simulink model "Modell_Entkopplung"  (R2025b)
settings: Solver=VariableStepAuto  StartTime=0.0  StopTime=10.0  RelTol=1e-3
values from neighbouring files (symbols this model uses):
  K1 = 4    [Modell_Entkopplung_Skript.m]
  K2 = 1    [Modell_Entkopplung_Skript.m]
  K3 = 3    [Modell_Entkopplung_Skript.m]
  K4 = 1    [Modell_Entkopplung_Skript.m]
  K5 = 1    [Modell_Entkopplung_Skript.m]
  K6 = 1    [Modell_Entkopplung_Skript.m]
  T1 = 1    [Modell_Entkopplung_Skript.m]
  T2 = 2    [Modell_Entkopplung_Skript.m]
  T3 = 1    [Modell_Entkopplung_Skript.m]
  T4 = 1    [Modell_Entkopplung_Skript.m]
  T5 = 1    [Modell_Entkopplung_Skript.m]
settings Model: Creator=ezech  LastModifiedBy=ezech

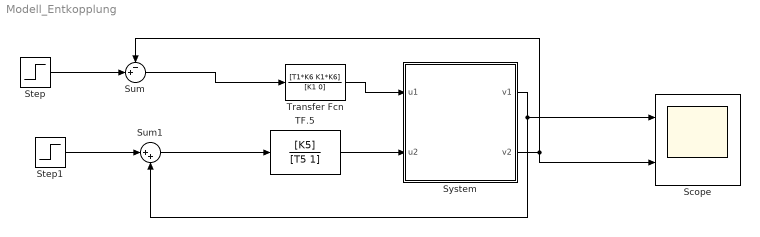
== system Modell_Entkopplung ==
  Scope : Scope  NumInputPorts=2
      settings: ActiveDisplayYMinimum=-1.0016844867769303  ActiveDisplayYMaximum=9.0151603809923753
  Step : Step  Time=0  SampleTime=0
  Step1 : Step  Time=0  After=0  SampleTime=0
  Sum : Sum  Inputs=-+|
  Sum1 : Sum  Inputs=|++
  System : Subsystem
  TF.5 : TransferFcn  Numerator=[K5]  Denominator=[T5 1]
  Transfer Fcn : TransferFcn  Numerator=[T1*K6 K1*K6]  Denominator=[K1 0]
  wires:
  Transfer Fcn/1 -> System/1(u1)
  TF.5/1 -> System/2(u2)
  Step/1 -> Sum/2
  System/2(v2) -> Sum/1, Scope/2
  Sum/1 -> Transfer Fcn/1
  Sum1/1 -> TF.5/1
  Step1/1 -> Sum1/1
  System/1(v1) -> Sum1/2, Scope/1

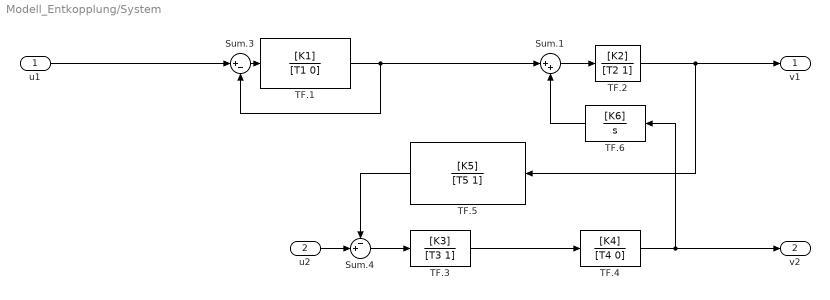
== system Modell_Entkopplung/System ==
  u1 : Inport
  u2 : Inport  Port=2
  Sum.1 : Sum  Inputs=|++  InputSameDT=on  SaturateOnIntegerOverflow=on  OutDataTypeStr=Inherit: Same as first input
  Sum.3 : Sum  Inputs=|+-  InputSameDT=on  SaturateOnIntegerOverflow=on  OutDataTypeStr=Inherit: Same as first input
  Sum.4 : Sum  Inputs=-+|  InputSameDT=on  SaturateOnIntegerOverflow=on  OutDataTypeStr=Inherit: Same as first input
  TF.1 : TransferFcn  Numerator=[K1]  Denominator=[T1 0]
  TF.2 : TransferFcn  Numerator=[K2]  Denominator=[T2 1]
  TF.3 : TransferFcn  Numerator=[K3]  Denominator=[T3 1]
  TF.4 : TransferFcn  Numerator=[K4]  Denominator=[T4 0]
  TF.5 : TransferFcn  Numerator=[K5]  Denominator=[T5 1]
  TF.6 : TransferFcn  Numerator=[K6]  Denominator=[1 0]
  v1 : Outport
  v2 : Outport  Port=2
  wires:
  TF.2/1 -> v1/1, TF.5/1
  TF.4/1 -> v2/1, TF.6/1
  TF.1/1 -> Sum.3/2, Sum.1/1
  Sum.1/1 -> TF.2/1
  TF.3/1 -> TF.4/1
  Sum.4/1 -> TF.3/1
  u2/1 -> Sum.4/2
  TF.5/1 -> Sum.4/1
  Sum.3/1 -> TF.1/1
  u1/1 -> Sum.3/1
  TF.6/1 -> Sum.1/2
